simulink model "ASM1_Influentmodel"  (Simulink 7.6)
settings: Solver=ode45  StartTime=0.0  StopTime=728.0  RelTol=1e-6
undefined symbols (not defined in the file or in its folder): aHpercent, CODpart_gperPEperd, CODpart_HH_max, CODpart_HH_min, CODpart_HH_ns, CODpart_HH_nv, CODpart_HH_st, CODpart_Ind_kgperd, CODpart_Ind_max, CODpart_Ind_min, CODpart_Ind_ns, CODpart_Ind_nv, CODpart_Ind_st, CODsol_gperPEperd, CODsol_HH_max, CODsol_HH_min, CODsol_HH_ns, CODsol_HH_nv, CODsol_HH_st, CODsol_Ind_kgperd, CODsol_Ind_max, CODsol_Ind_min, CODsol_Ind_ns, CODsol_Ind_nv, CODsol_Ind_st, FFfraction, HHnoiseswitch, HHpolnoiseswitch, HHpopswitch, Indnoiseswitch, Indpolnoiseswitch, Indpopswitch, InfAmp, InfBias, Infcst, InfFreq, InfPhase, LLrain, PE, polnoiseswitch, Q_HH_ns, Q_HH_nv, Q_HH_st, Q_Ind_ns, Q_Ind_nv, Q_Ind_st, Q_SCI_ns, Q_SCI_nv, Q_SCI_st, QHHsatmax, QHHsatmin, QInd_weekday, QIndsatmax, QIndsatmin, Qpermm, QperPE, QSCIsatmax, QSCIsatmin, rain_nm, rain_ns ... (+85)
libraries: simulink x5
Description:
  | BSM2 influent model, version 15 March 2005
settings Model: Creator=Krist V. Gernaey  LastModifiedBy=xavier  ExtModeAutoUpdateStatusClock=off
settings DataIOCC: LimitDataPoints=off  SignalLoggingName=sigsOut  OutputOption=SpecifiedOutputTimes  OutputTimes=[119.0:1.0/96.0:728.0]
settings OptimizationCC: InitFltsAndDblsToZero=on
settings DebuggingCC: SaveWithParameterizedLinksMsg=none  SignalResolutionControl=TryResolveAllWithWarning  SolverPrmCheckMsg=none  MultiTaskDSMMsg=warning  MultiTaskCondExecSysMsg=none  StrictBusMsg=None
settings HardwareCC: TargetEndianess=LittleEndian  TargetHWDeviceType=MATLAB Host  ProdEqTarget=off
settings RTWCC: IncludeERTFirstTime=on

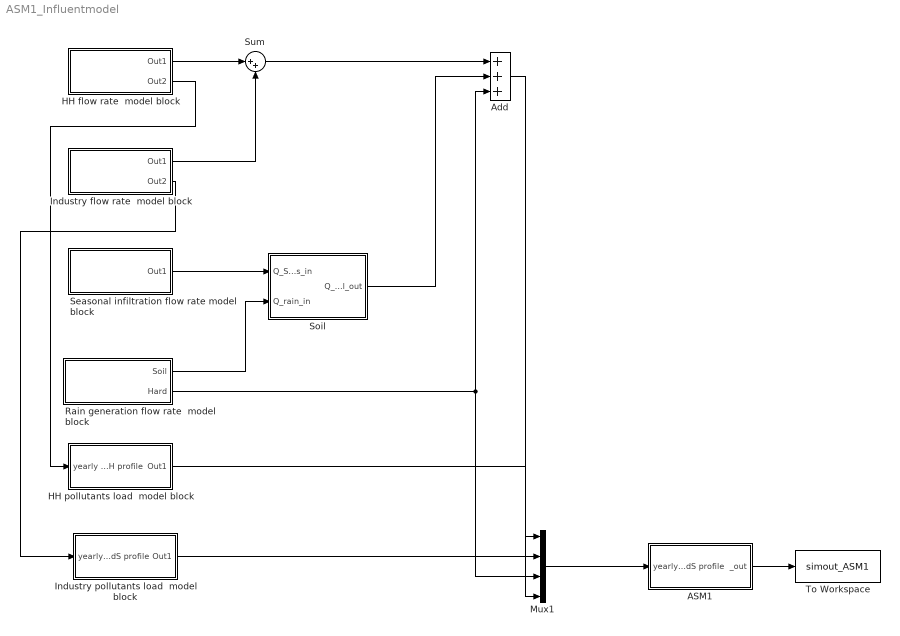
== system ASM1_Influentmodel ==
  ASM1 : Subsystem
  Add : Sum  Inputs=+++
  HH flow rate  model block : Subsystem
  "HH pollutants load  model block " : Subsystem
  Industry flow rate  model block : Subsystem
  "Industry pollutants load  model block " : Subsystem
  Mux1 : Mux
  Rain generation flow rate  model block : Subsystem
  Seasonal infiltration flow rate model block : Subsystem
  Soil : Subsystem
  Sum : Sum  Inputs=|++  SaturateOnIntegerOverflow=on
  To Workspace : ToWorkspace  VariableName=simout_ASM1  SampleTime=-1  SaveFormat=Array
  wires:
  Add/1 -> Mux1/4
  Rain generation flow rate  model block/2(Hard) -> Mux1/3, Add/3
  Soil/1(Q_Soil_out) -> Add/2
  Sum/1 -> Add/1
  HH flow rate  model block/1(Out1) -> Sum/1
  Rain generation flow rate  model block/1(Soil) -> Soil/2(Q_rain_in)
  Seasonal infiltration flow rate model block/1(Out1) -> Soil/1(Q_Seas_in)
  Industry flow rate  model block/1(Out1) -> Sum/2
  HH flow rate  model block/2(Out2) -> "HH pollutants load  model block "/1(yearly HH profile)
  Industry flow rate  model block/2(Out2) -> "Industry pollutants load  model block "/1(yearly_indS profile)
  "HH pollutants load  model block "/1(Out1) -> Mux1/1
  "Industry pollutants load  model block "/1(Out1) -> Mux1/2
  Mux1/1 -> ASM1/1(yearly_indS profile)
  ASM1/1(_out) -> To Workspace/1

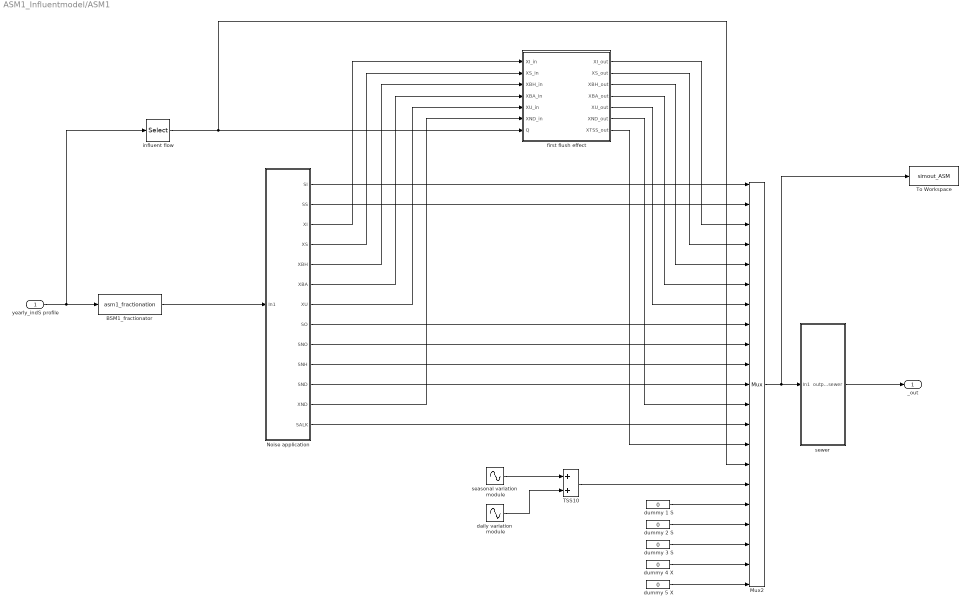
== system ASM1_Influentmodel/ASM1 ==
  yearly_indS profile : Inport
  BSM1_fractionator : S-Function  FunctionName=asm1_fractionation  Parameters=ASM1_PARS, ASM1_FRACTIONS  EnableBusSupport=off
  Mux2 : Mux  Inputs=21
  Noise application : Subsystem
  TSS10 : Sum
  To Workspace : ToWorkspace  VariableName=simout_ASM  SampleTime=-1  SaveFormat=Array
  daily variation  module : Sin  Amplitude=TdAmp  Bias=TdBias  Frequency=TdFreq  Phase=TdPhase  SampleTime=0
  dummy 1 S : Constant  Value=0
  dummy 2 S : Constant  Value=0
  dummy 3 S : Constant  Value=0
  dummy 4 X : Constant  Value=0
  dummy 5 X : Constant  Value=0
  first flush effect : Subsystem
  influent flow : Selector  InputPortWidth=12  IndexOptions=Index vector (dialog)  Indices=[12]  OutputSizes=1
  seasonal variation  module : Sin  Amplitude=TAmp  Bias=TBias  Frequency=TFreq  Phase=TPhase  SampleTime=0
  sewer : Subsystem
  _out : Outport
  wires:
  yearly_indS profile/1 -> influent flow/1, BSM1_fractionator/1
  BSM1_fractionator/1 -> Noise application/1(In1)
  Noise application/3(XI) -> first flush effect/1(XI_in)
  Noise application/4(XS) -> first flush effect/2(XS_in)
  Noise application/5(XBH) -> first flush effect/3(XBH_in)
  Noise application/6(XBA) -> first flush effect/4(XBA_in)
  Noise application/7(XU) -> first flush effect/5(XU_in)
  Noise application/12(XND) -> first flush effect/6(XND_in)
  influent flow/1 -> first flush effect/7(Q), Mux2/15
  Mux2/1 -> sewer/1(In1), To Workspace/1
  sewer/1(output sewer) -> _out/1
  dummy 5 X/1 -> Mux2/21
  dummy 4 X/1 -> Mux2/20
  dummy 3 S/1 -> Mux2/19
  dummy 2 S/1 -> Mux2/18
  dummy 1 S/1 -> Mux2/17
  Noise application/2(SS) -> Mux2/2
  Noise application/1(SI) -> Mux2/1
  first flush effect/1(XI_out) -> Mux2/3
  first flush effect/2(XS_out) -> Mux2/4
  first flush effect/3(XBH_out) -> Mux2/5
  first flush effect/4(XBA_out) -> Mux2/6
  first flush effect/5(XU_out) -> Mux2/7
  Noise application/8(SO) -> Mux2/8
  Noise application/9(SNO) -> Mux2/9
  Noise application/10(SNH) -> Mux2/10
  Noise application/11(SND) -> Mux2/11
  first flush effect/6(XND_out) -> Mux2/12
  Noise application/13(SALK) -> Mux2/13
  first flush effect/7(XTSS_out) -> Mux2/14
  seasonal variation  module/1 -> TSS10/1
  daily variation  module/1 -> TSS10/2
  TSS10/1 -> Mux2/16

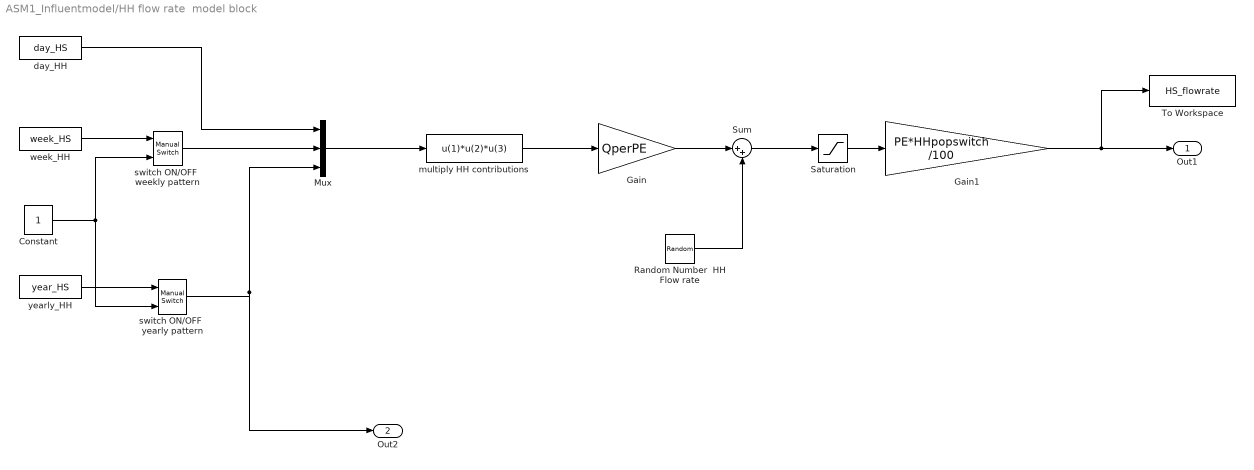
== system ASM1_Influentmodel/HH flow rate  model block ==
  Constant : Constant
  Gain : Gain  Gain=QperPE
  Gain1 : Gain  Gain=PE*HHpopswitch /100
  Mux : Mux  Inputs=3
  Random Number  HH Flow rate : RandomNumber  Variance=Q_HH_nv*HHnoiseswitch  Seed=Q_HH_ns  SampleTime=Q_HH_st
  Saturation : Saturate  UpperLimit=QHHsatmax  LowerLimit=QHHsatmin
  Sum : Sum  Inputs=|++
  To Workspace : ToWorkspace  VariableName=HS_flowrate  SampleTime=-1  SaveFormat=Array
  day_HH : FromWorkspace  VariableName=day_HS  SampleTime=1/24  Interpolate=off  OutputAfterFinalValue=Cyclic repetition
  multiply HH contributions : Fcn  Expr=u(1)*u(2)*u(3)
  switch ON/OFF  weekly pattern : simulink/Signal Routing/Manual Switch  SystemSampleTime=-1  sw=1  action=0  varsize=off
  switch ON/OFF  yearly pattern : simulink/Signal Routing/Manual Switch  SystemSampleTime=-1  sw=1  action=0  varsize=off
  week_HH : FromWorkspace  VariableName=week_HS  SampleTime=1  Interpolate=off  OutputAfterFinalValue=Cyclic repetition
  yearly_HH : FromWorkspace  VariableName=year_HS  SampleTime=1  Interpolate=off  OutputAfterFinalValue=Cyclic repetition
  Out1 : Outport
  Out2 : Outport  Port=2
  wires:
  multiply HH contributions/1 -> Gain/1
  Gain/1 -> Sum/1
  Saturation/1 -> Gain1/1
  Gain1/1 -> Out1/1, To Workspace/1
  Random Number  HH Flow rate/1 -> Sum/2
  week_HH/1 -> switch ON/OFF  weekly pattern/1
  yearly_HH/1 -> switch ON/OFF  yearly pattern/1
  day_HH/1 -> Mux/1
  switch ON/OFF  weekly pattern/1 -> Mux/2
  switch ON/OFF  yearly pattern/1 -> Mux/3, Out2/1
  Constant/1 -> switch ON/OFF  weekly pattern/2, switch ON/OFF  yearly pattern/2
  Mux/1 -> multiply HH contributions/1
  Sum/1 -> Saturation/1

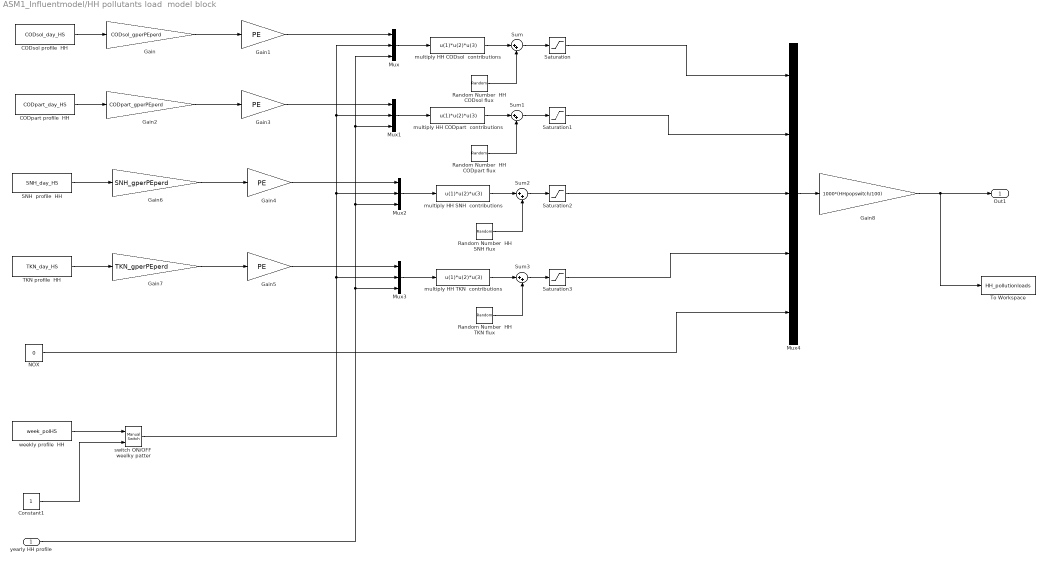
== system ASM1_Influentmodel/HH pollutants load  model block  ==
  yearly HH profile : Inport
  CODpart profile  HH : FromWorkspace  VariableName=CODpart_day_HS  SampleTime=1/24  Interpolate=off  OutputAfterFinalValue=Cyclic repetition
  CODsol profile  HH : FromWorkspace  VariableName=CODsol_day_HS  SampleTime=1/24  Interpolate=off  OutputAfterFinalValue=Cyclic repetition
  Constant1 : Constant
  Gain : Gain  Gain=CODsol_gperPEperd
  Gain{1,3..5} (4 alike) : Gain  Gain=PE
  Gain2 : Gain  Gain=CODpart_gperPEperd
  Gain6 : Gain  Gain=SNH_gperPEperd
  Gain7 : Gain  Gain=TKN_gperPEperd
  Gain8 : Gain  Gain=1000*(HHpopswitch/100)
  Mux{,1..3} (4 alike) : Mux  Inputs=3
  Mux4 : Mux  Inputs=5
  NOX : Constant  Value=0
  Random Number  HH CODpart flux : RandomNumber  Variance=CODpart_HH_nv*HHpolnoiseswitch  Seed=CODpart_HH_ns  SampleTime=CODpart_HH_st
  Random Number  HH CODsol flux : RandomNumber  Variance=CODsol_HH_nv*HHpolnoiseswitch  Seed=CODsol_HH_ns  SampleTime=CODsol_HH_st
  Random Number  HH SNH flux : RandomNumber  Variance=SNH_HH_nv*HHpolnoiseswitch  Seed=SNH_HH_ns  SampleTime=SNH_HH_st
  Random Number  HH TKN flux : RandomNumber  Variance=TKN_HH_nv*HHpolnoiseswitch  Seed=TKN_HH_ns  SampleTime=TKN_HH_st
  SNH  profile  HH : FromWorkspace  VariableName=SNH_day_HS  SampleTime=1/24  Interpolate=off  OutputAfterFinalValue=Cyclic repetition
  Saturation : Saturate  UpperLimit=CODsol_HH_max  LowerLimit=CODsol_HH_min
  Saturation1 : Saturate  UpperLimit=CODpart_HH_max  LowerLimit=CODpart_HH_min
  Saturation2 : Saturate  UpperLimit=SNH_HH_max  LowerLimit=SNH_HH_min
  Saturation3 : Saturate  UpperLimit=TKN_HH_max  LowerLimit=TKN_HH_min
  Sum{,1..3} (4 alike) : Sum  Inputs=|++
  TKN profile  HH : FromWorkspace  VariableName=TKN_day_HS  SampleTime=1/24  Interpolate=off  OutputAfterFinalValue=Cyclic repetition
  To Workspace : ToWorkspace  VariableName=HH_pollutionloads  SampleTime=-1  SaveFormat=Array
  multiply HH CODpart  contributions : Fcn  Expr=u(1)*u(2)*u(3)
  multiply HH CODsol  contributions : Fcn  Expr=u(1)*u(2)*u(3)
  multiply HH SNH  contributions : Fcn  Expr=u(1)*u(2)*u(3)
  multiply HH TKN  contributions : Fcn  Expr=u(1)*u(2)*u(3)
  switch ON/OFF  weelky patter : simulink/Signal Routing/Manual Switch  SystemSampleTime=-1  sw=1  action=0  varsize=off
  weekly profile  HH : FromWorkspace  VariableName=week_polHS  SampleTime=1  Interpolate=off  OutputAfterFinalValue=Cyclic repetition
  Out1 : Outport
  wires:
  Random Number  HH CODsol flux/1 -> Sum/2
  CODsol profile  HH/1 -> Gain/1
  Gain/1 -> Gain1/1
  Mux/1 -> multiply HH CODsol  contributions/1
  multiply HH CODsol  contributions/1 -> Sum/1
  Sum/1 -> Saturation/1
  Gain1/1 -> Mux/1
  Random Number  HH CODpart flux/1 -> Sum1/2
  CODpart profile  HH/1 -> Gain2/1
  Gain2/1 -> Gain3/1
  Mux1/1 -> multiply HH CODpart  contributions/1
  multiply HH CODpart  contributions/1 -> Sum1/1
  Sum1/1 -> Saturation1/1
  Gain3/1 -> Mux1/1
  Random Number  HH SNH flux/1 -> Sum2/2
  SNH  profile  HH/1 -> Gain6/1
  Gain6/1 -> Gain4/1
  Mux2/1 -> multiply HH SNH  contributions/1
  multiply HH SNH  contributions/1 -> Sum2/1
  Sum2/1 -> Saturation2/1
  Gain4/1 -> Mux2/1
  Random Number  HH TKN flux/1 -> Sum3/2
  TKN profile  HH/1 -> Gain7/1
  Gain7/1 -> Gain5/1
  Mux3/1 -> multiply HH TKN  contributions/1
  multiply HH TKN  contributions/1 -> Sum3/1
  Sum3/1 -> Saturation3/1
  Gain5/1 -> Mux3/1
  Mux4/1 -> Gain8/1
  Constant1/1 -> switch ON/OFF  weelky patter/2
  weekly profile  HH/1 -> switch ON/OFF  weelky patter/1
  Saturation/1 -> Mux4/1
  Saturation1/1 -> Mux4/2
  Saturation2/1 -> Mux4/3
  Saturation3/1 -> Mux4/4
  NOX/1 -> Mux4/5
  switch ON/OFF  weelky patter/1 -> Mux2/2, Mux/2, Mux1/2, Mux3/2
  yearly HH profile/1 -> Mux2/3, Mux/3, Mux1/3, Mux3/3
  Gain8/1 -> Out1/1, To Workspace/1

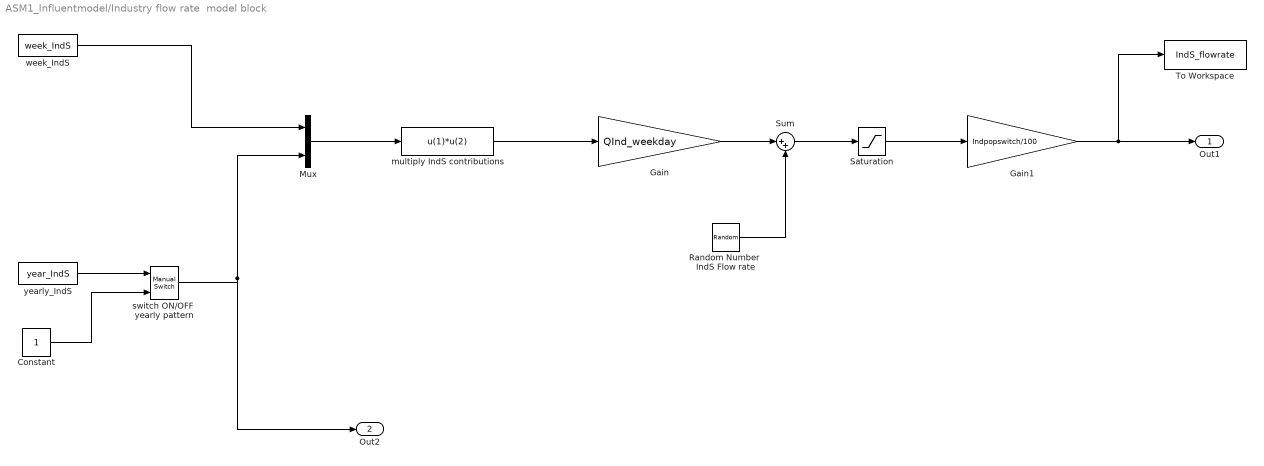
== system ASM1_Influentmodel/Industry flow rate  model block ==
  Constant : Constant
  Gain : Gain  Gain=QInd_weekday
  Gain1 : Gain  Gain=Indpopswitch/100
  Mux : Mux  Inputs=2
  Random Number  IndS Flow rate : RandomNumber  Variance=Q_Ind_nv*Indnoiseswitch  Seed=Q_Ind_ns  SampleTime=Q_Ind_st
  Saturation : Saturate  UpperLimit=QIndsatmax  LowerLimit=QIndsatmin
  Sum : Sum  Inputs=|++
  To Workspace : ToWorkspace  VariableName=IndS_flowrate  SampleTime=-1  SaveFormat=Array
  multiply IndS contributions : Fcn  Expr=u(1)*u(2)
  switch ON/OFF  yearly pattern : simulink/Signal Routing/Manual Switch  SystemSampleTime=-1  sw=1  action=0  varsize=off
  week_IndS : FromWorkspace  VariableName=week_IndS  SampleTime=1/6  Interpolate=off  OutputAfterFinalValue=Cyclic repetition
  yearly_IndS : FromWorkspace  VariableName=year_IndS  SampleTime=1  Interpolate=off  OutputAfterFinalValue=Cyclic repetition
  Out1 : Outport
  Out2 : Outport  Port=2
  wires:
  multiply IndS contributions/1 -> Gain/1
  Gain/1 -> Sum/1
  Sum/1 -> Saturation/1
  Saturation/1 -> Gain1/1
  Gain1/1 -> Out1/1, To Workspace/1
  Random Number  IndS Flow rate/1 -> Sum/2
  yearly_IndS/1 -> switch ON/OFF  yearly pattern/1
  week_IndS/1 -> Mux/1
  switch ON/OFF  yearly pattern/1 -> Mux/2, Out2/1
  Constant/1 -> switch ON/OFF  yearly pattern/2
  Mux/1 -> multiply IndS contributions/1

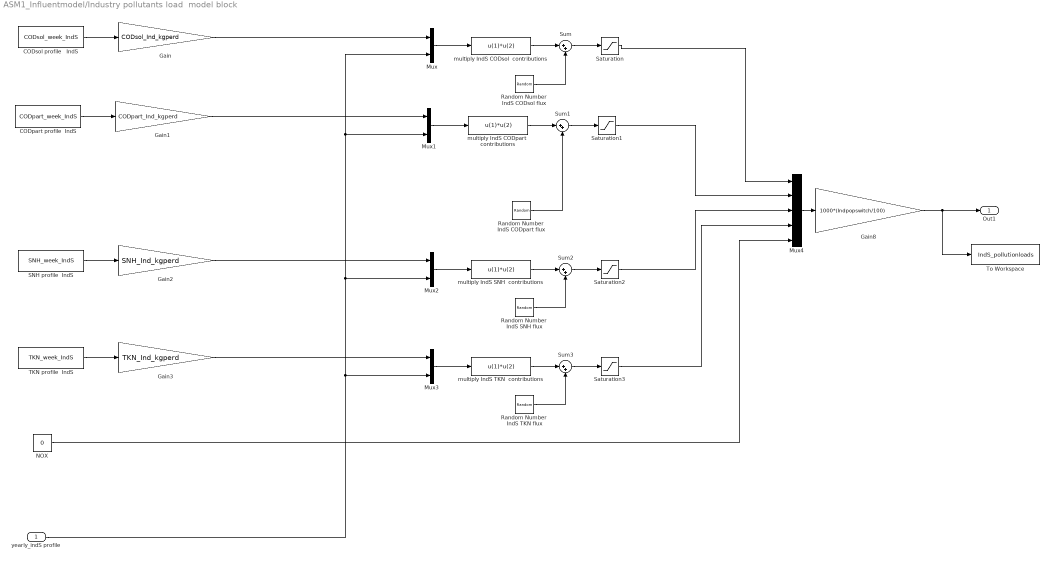
== system ASM1_Influentmodel/Industry pollutants load  model block  ==
  yearly_indS profile : Inport
  CODpart profile  IndS : FromWorkspace  VariableName=CODpart_week_IndS  SampleTime=1/6  Interpolate=off  OutputAfterFinalValue=Cyclic repetition
  CODsol profile   IndS : FromWorkspace  VariableName=CODsol_week_IndS  SampleTime=1/6  Interpolate=off  OutputAfterFinalValue=Cyclic repetition
  Gain : Gain  Gain=CODsol_Ind_kgperd
  Gain1 : Gain  Gain=CODpart_Ind_kgperd
  Gain2 : Gain  Gain=SNH_Ind_kgperd
  Gain3 : Gain  Gain=TKN_Ind_kgperd
  Gain8 : Gain  Gain=1000*(Indpopswitch/100)
  Mux{,1..3} (4 alike) : Mux  Inputs=2
  Mux4 : Mux  Inputs=5
  NOX : Constant  Value=0
  Random Number  IndS CODpart flux : RandomNumber  Variance=CODpart_Ind_nv*Indpolnoiseswitch  Seed=CODpart_Ind_ns  SampleTime=CODpart_Ind_st
  Random Number  IndS CODsol flux : RandomNumber  Variance=CODsol_Ind_nv*Indpolnoiseswitch  Seed=CODsol_Ind_ns  SampleTime=CODsol_Ind_st
  Random Number  IndS SNH flux : RandomNumber  Variance=SNH_Ind_nv*Indpolnoiseswitch  Seed=SNH_Ind_ns  SampleTime=SNH_Ind_st
  Random Number  IndS TKN flux : RandomNumber  Variance=TKN_Ind_nv*Indpolnoiseswitch  Seed=TKN_Ind_ns  SampleTime=TKN_Ind_st
  SNH profile  IndS : FromWorkspace  VariableName=SNH_week_IndS  SampleTime=1/6  Interpolate=off  OutputAfterFinalValue=Cyclic repetition
  Saturation : Saturate  UpperLimit=CODsol_Ind_max  LowerLimit=CODsol_Ind_min
  Saturation1 : Saturate  UpperLimit=CODpart_Ind_max  LowerLimit=CODpart_Ind_min
  Saturation2 : Saturate  UpperLimit=SNH_Ind_max  LowerLimit=SNH_Ind_min
  Saturation3 : Saturate  UpperLimit=TKN_Ind_max  LowerLimit=TKN_Ind_min
  Sum{,1..3} (4 alike) : Sum  Inputs=|++
  TKN profile  IndS : FromWorkspace  VariableName=TKN_week_IndS  SampleTime=1/6  Interpolate=off  OutputAfterFinalValue=Cyclic repetition
  To Workspace : ToWorkspace  VariableName=IndS_pollutionloads  SampleTime=-1  SaveFormat=Array
  multiply IndS CODpart  contributions : Fcn  Expr=u(1)*u(2)
  multiply IndS CODsol  contributions : Fcn  Expr=u(1)*u(2)
  multiply IndS SNH  contributions : Fcn  Expr=u(1)*u(2)
  multiply IndS TKN  contributions : Fcn  Expr=u(1)*u(2)
  Out1 : Outport
  wires:
  Random Number  IndS CODsol flux/1 -> Sum/2
  CODsol profile   IndS/1 -> Gain/1
  Mux/1 -> multiply IndS CODsol  contributions/1
  multiply IndS CODsol  contributions/1 -> Sum/1
  Sum/1 -> Saturation/1
  Mux4/1 -> Gain8/1
  Gain/1 -> Mux/1
  Random Number  IndS CODpart flux/1 -> Sum1/2
  CODpart profile  IndS/1 -> Gain1/1
  Mux1/1 -> multiply IndS CODpart  contributions/1
  multiply IndS CODpart  contributions/1 -> Sum1/1
  Sum1/1 -> Saturation1/1
  Gain1/1 -> Mux1/1
  Random Number  IndS SNH flux/1 -> Sum2/2
  SNH profile  IndS/1 -> Gain2/1
  Mux2/1 -> multiply IndS SNH  contributions/1
  multiply IndS SNH  contributions/1 -> Sum2/1
  Sum2/1 -> Saturation2/1
  Gain2/1 -> Mux2/1
  Random Number  IndS TKN flux/1 -> Sum3/2
  TKN profile  IndS/1 -> Gain3/1
  Mux3/1 -> multiply IndS TKN  contributions/1
  multiply IndS TKN  contributions/1 -> Sum3/1
  Sum3/1 -> Saturation3/1
  Gain3/1 -> Mux3/1
  yearly_indS profile/1 -> Mux3/2, Mux2/2, Mux/2, Mux1/2
  Saturation/1 -> Mux4/1
  Saturation1/1 -> Mux4/2
  Saturation2/1 -> Mux4/3
  Saturation3/1 -> Mux4/4
  NOX/1 -> Mux4/5
  Gain8/1 -> Out1/1, To Workspace/1

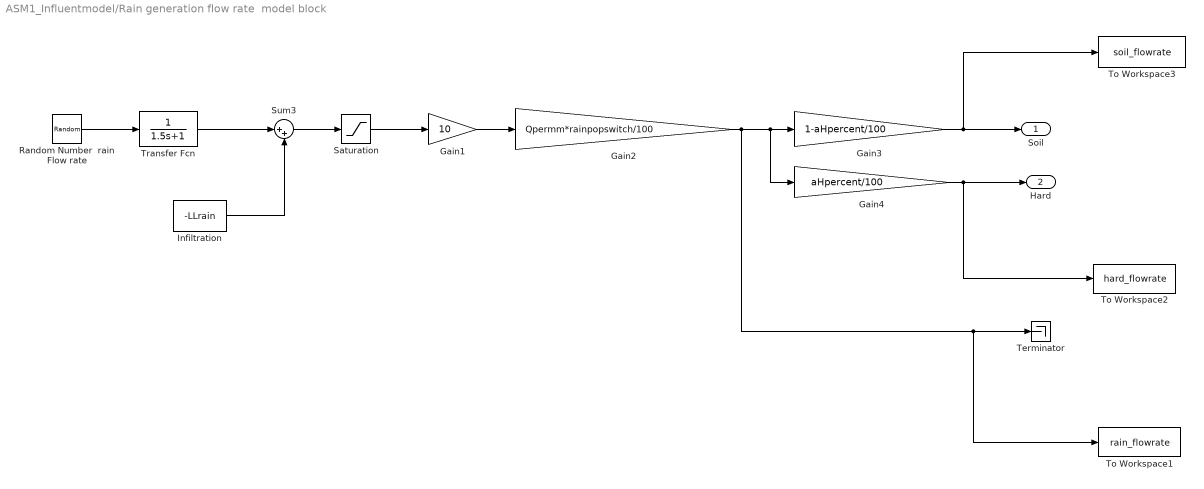
== system ASM1_Influentmodel/Rain generation flow rate  model block ==
  Gain1 : Gain  Gain=10  SaturateOnIntegerOverflow=on  OutDataTypeStr=Inherit: Same as input  ParamDataTypeStr=Inherit: Same as input
  Gain2 : Gain  Gain=Qpermm*rainpopswitch/100  SaturateOnIntegerOverflow=on  OutDataTypeStr=Inherit: Same as input  ParamDataTypeStr=Inherit: Same as input
  Gain3 : Gain  Gain=1-aHpercent/100  SaturateOnIntegerOverflow=on  OutDataTypeStr=Inherit: Same as input  ParamDataTypeStr=Inherit: Same as input
  Gain4 : Gain  Gain=aHpercent/100  SaturateOnIntegerOverflow=on  OutDataTypeStr=Inherit: Same as input  ParamDataTypeStr=Inherit: Same as input
  Infiltration : Constant  Value=-LLrain
  Random Number  rain Flow rate : RandomNumber  Mean=rain_nm  Variance=rain_nv  Seed=rain_ns  SampleTime=rain_st
  Saturation : Saturate  UpperLimit=rainmax  LowerLimit=rainmin
  Sum3 : Sum  Inputs=|++  SaturateOnIntegerOverflow=on
  Terminator : Terminator
  To Workspace1 : ToWorkspace  VariableName=rain_flowrate  SampleTime=-1  SaveFormat=Array
  To Workspace2 : ToWorkspace  VariableName=hard_flowrate  SampleTime=-1  SaveFormat=Array
  To Workspace3 : ToWorkspace  VariableName=soil_flowrate  SampleTime=-1  SaveFormat=Array
  Transfer Fcn : TransferFcn  Denominator=[1.5 1]
  Soil : Outport
  Hard : Outport  Port=2
  wires:
  Random Number  rain Flow rate/1 -> Transfer Fcn/1
  Gain3/1 -> Soil/1, To Workspace3/1
  Gain4/1 -> Hard/1, To Workspace2/1
  Gain2/1 -> Gain4/1, Gain3/1, To Workspace1/1, Terminator/1
  Gain1/1 -> Gain2/1
  Saturation/1 -> Gain1/1
  Infiltration/1 -> Sum3/2
  Transfer Fcn/1 -> Sum3/1
  Sum3/1 -> Saturation/1

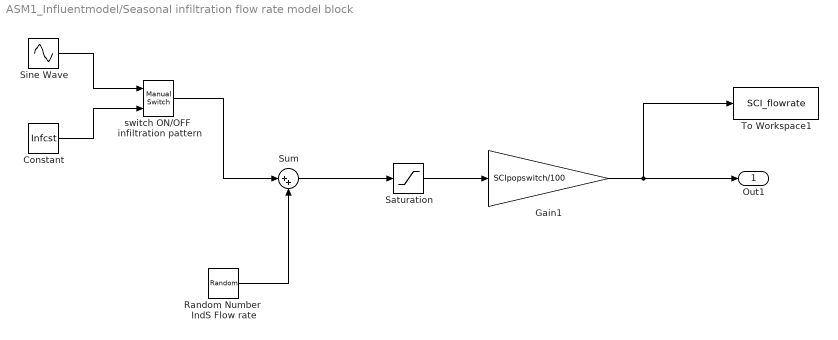
== system ASM1_Influentmodel/Seasonal infiltration flow rate model block ==
  Constant : Constant  Value=Infcst
  Gain1 : Gain  Gain=SCIpopswitch/100
  Random Number  IndS Flow rate : RandomNumber  Variance=Q_SCI_nv*SCInoiseswitch  Seed=Q_SCI_ns  SampleTime=Q_SCI_st
  Saturation : Saturate  UpperLimit=QSCIsatmax  LowerLimit=QSCIsatmin
  Sine Wave : Sin  Amplitude=InfAmp  Bias=InfBias  Frequency=InfFreq  Phase=InfPhase  SampleTime=0
  Sum : Sum  Inputs=|++
  To Workspace1 : ToWorkspace  VariableName=SCI_flowrate  SampleTime=-1  SaveFormat=Array
  switch ON/OFF  infiltration pattern : simulink/Signal Routing/Manual Switch  SystemSampleTime=-1  sw=1  action=0  varsize=off
  Out1 : Outport
  wires:
  switch ON/OFF  infiltration pattern/1 -> Sum/1
  Sum/1 -> Saturation/1
  Saturation/1 -> Gain1/1
  Gain1/1 -> Out1/1, To Workspace1/1
  Random Number  IndS Flow rate/1 -> Sum/2
  Sine Wave/1 -> switch ON/OFF  infiltration pattern/1
  Constant/1 -> switch ON/OFF  infiltration pattern/2

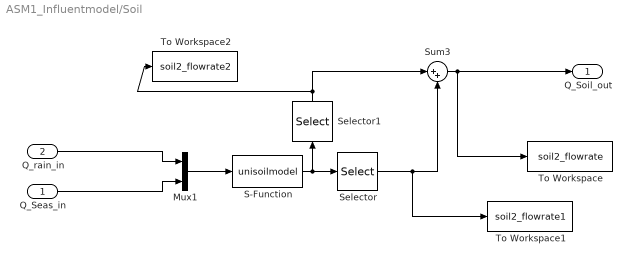
== system ASM1_Influentmodel/Soil ==
  Q_Seas_in : Inport
  Q_rain_in : Inport  Port=2
  Mux1 : Mux  Inputs=2
  S-Function : S-Function  FunctionName=unisoilmodel  Parameters=XINITSOIL, PARS_SOIL  EnableBusSupport=off
  Selector : Selector  InputPortWidth=4  IndexOptions=Index vector (dialog)  Indices=[1]  OutputSizes=1
  Selector1 : Selector  InputPortWidth=4  IndexOptions=Index vector (dialog)  Indices=[2]  OutputSizes=1
  Sum3 : Sum  Inputs=|++  SaturateOnIntegerOverflow=on
  To Workspace : ToWorkspace  VariableName=soil2_flowrate  SampleTime=-1  SaveFormat=Array
  To Workspace1 : ToWorkspace  VariableName=soil2_flowrate1  SampleTime=-1  SaveFormat=Array
  To Workspace2 : ToWorkspace  VariableName=soil2_flowrate2  SampleTime=-1  SaveFormat=Array
  Q_Soil_out : Outport
  wires:
  S-Function/1 -> Selector/1, Selector1/1
  Selector1/1 -> Sum3/1, To Workspace2/1
  Selector/1 -> Sum3/2, To Workspace1/1
  Sum3/1 -> Q_Soil_out/1, To Workspace/1
  Mux1/1 -> S-Function/1
  Q_rain_in/1 -> Mux1/1
  Q_Seas_in/1 -> Mux1/2

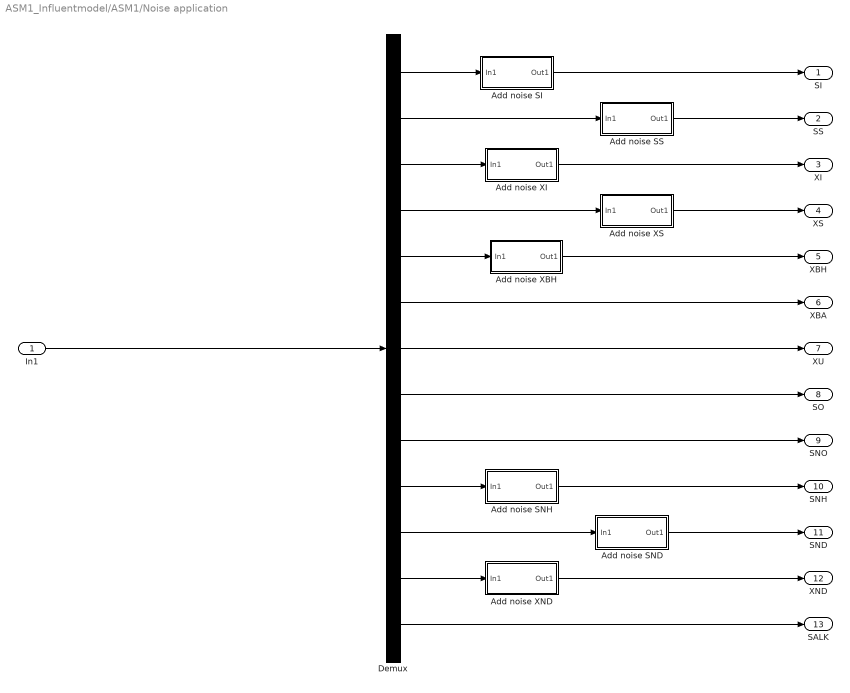
== system ASM1_Influentmodel/ASM1/Noise application ==
  In1 : Inport
  Add noise SI : Subsystem
  Add noise SND : Subsystem
  Add noise SNH : Subsystem
  Add noise SS : Subsystem
  Add noise XBH : Subsystem
  Add noise XI : Subsystem
  Add noise XND : Subsystem
  Add noise XS : Subsystem
  Demux : Demux  Outputs=[1 1 1 1 1 1 1 1 1 1 1 1 1]
  SI : Outport
  SS : Outport  Port=2
  XI : Outport  Port=3
  XS : Outport  Port=4
  XBH : Outport  Port=5
  XBA : Outport  Port=6
  XU : Outport  Port=7
  SO : Outport  Port=8
  SNO : Outport  Port=9
  SNH : Outport  Port=10
  SND : Outport  Port=11
  XND : Outport  Port=12
  SALK : Outport  Port=13
  wires:
  In1/1 -> Demux/1
  Demux/1 -> Add noise SI/1(In1)
  Demux/2 -> Add noise SS/1(In1)
  Demux/3 -> Add noise XI/1(In1)
  Demux/4 -> Add noise XS/1(In1)
  Demux/5 -> Add noise XBH/1(In1)
  Demux/6 -> XBA/1
  Demux/7 -> XU/1
  Demux/8 -> SO/1
  Demux/9 -> SNO/1
  Demux/10 -> Add noise SNH/1(In1)
  Demux/11 -> Add noise SND/1(In1)
  Demux/12 -> Add noise XND/1(In1)
  Demux/13 -> SALK/1
  Add noise SI/1(Out1) -> SI/1
  Add noise SS/1(Out1) -> SS/1
  Add noise XI/1(Out1) -> XI/1
  Add noise XS/1(Out1) -> XS/1
  Add noise XBH/1(Out1) -> XBH/1
  Add noise SNH/1(Out1) -> SNH/1
  Add noise SND/1(Out1) -> SND/1
  Add noise XND/1(Out1) -> XND/1

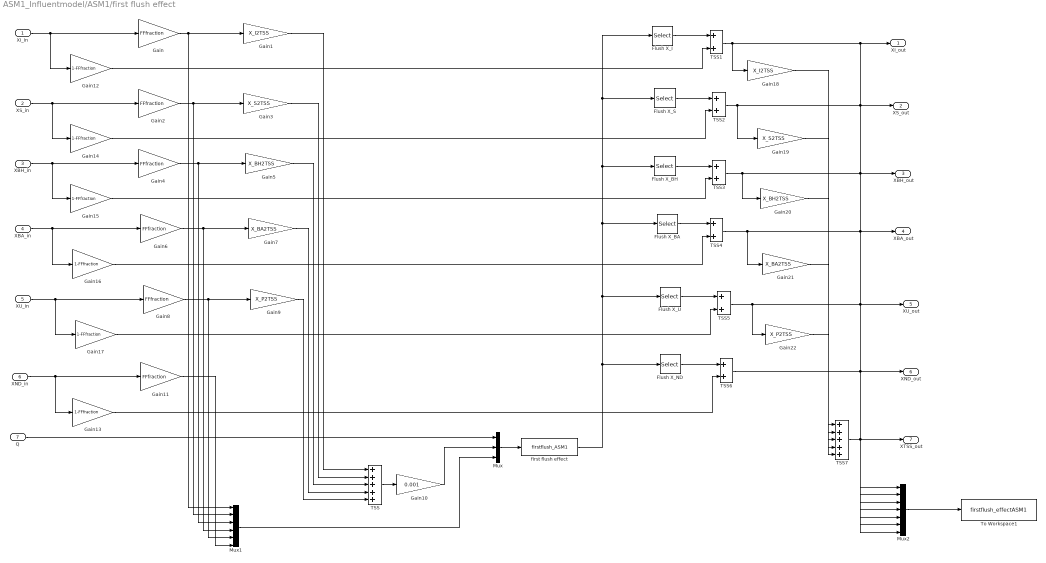
== system ASM1_Influentmodel/ASM1/first flush effect ==
  XI_in : Inport
  XS_in : Inport  Port=2
  XBH_in : Inport  Port=3
  XBA_in : Inport  Port=4
  XU_in : Inport  Port=5
  XND_in : Inport  Port=6
  Q : Inport  Port=7
  Flush X_BA : Selector  InputPortWidth=15  IndexOptions=Index vector (dialog)  Indices=[6]  OutputSizes=1
  Flush X_BH : Selector  InputPortWidth=15  IndexOptions=Index vector (dialog)  Indices=[5]  OutputSizes=1
  Flush X_I : Selector  InputPortWidth=15  IndexOptions=Index vector (dialog)  Indices=[3]  OutputSizes=1
  Flush X_ND : Selector  InputPortWidth=15  IndexOptions=Index vector (dialog)  Indices=[8]  OutputSizes=1
  Flush X_S : Selector  InputPortWidth=15  IndexOptions=Index vector (dialog)  Indices=[4]  OutputSizes=1
  Flush X_U : Selector  InputPortWidth=15  IndexOptions=Index vector (dialog)  Indices=[7]  OutputSizes=1
  Gain{,2,4,6,8,11} (6 alike) : Gain  Gain=FFfraction
  Gain1 : Gain  Gain=X_I2TSS
  Gain10 : Gain  Gain=0.001
  Gain{12..17} (6 alike) : Gain  Gain=1-FFfraction
  Gain18 : Gain  Gain=X_I2TSS
  Gain19 : Gain  Gain=X_S2TSS
  Gain20 : Gain  Gain=X_BH2TSS
  Gain21 : Gain  Gain=X_BA2TSS
  Gain22 : Gain  Gain=X_P2TSS
  Gain3 : Gain  Gain=X_S2TSS
  Gain5 : Gain  Gain=X_BH2TSS
  Gain7 : Gain  Gain=X_BA2TSS
  Gain9 : Gain  Gain=X_P2TSS
  Mux : Mux  Inputs=3
  Mux1 : Mux  Inputs=6
  Mux2 : Mux  Inputs=7
  TSS : Sum  Inputs=+++++
  TSS{1..6} (6 alike) : Sum
  TSS7 : Sum  Inputs=+++++
  To Workspace1 : ToWorkspace  VariableName=firstflush_effectASM1  SampleTime=-1  SaveFormat=Array
  first flush effect : S-Function  FunctionName=firstflush_ASM1  Parameters=ASM1_XINIT, SSPARS  EnableBusSupport=off
  XI_out : Outport
  XS_out : Outport  Port=2
  XBH_out : Outport  Port=3
  XBA_out : Outport  Port=4
  XU_out : Outport  Port=5
  XND_out : Outport  Port=6
  XTSS_out : Outport  Port=7
  wires:
  XI_in/1 -> Gain/1, Gain12/1
  Gain/1 -> Gain1/1, Mux1/1
  XS_in/1 -> Gain2/1, Gain14/1
  Gain2/1 -> Gain3/1, Mux1/2
  XBH_in/1 -> Gain4/1, Gain15/1
  Gain4/1 -> Gain5/1, Mux1/3
  XBA_in/1 -> Gain6/1, Gain16/1
  Gain6/1 -> Gain7/1, Mux1/4
  XU_in/1 -> Gain8/1, Gain17/1
  Gain8/1 -> Gain9/1, Mux1/5
  Gain1/1 -> TSS/1
  Gain3/1 -> TSS/2
  Gain5/1 -> TSS/3
  Gain7/1 -> TSS/4
  Gain9/1 -> TSS/5
  Mux1/1 -> Mux/3
  Gain11/1 -> Mux1/6
  XND_in/1 -> Gain11/1, Gain13/1
  Q/1 -> Mux/1
  Mux/1 -> first flush effect/1
  TSS/1 -> Gain10/1
  Gain10/1 -> Mux/2
  Gain12/1 -> TSS1/2
  first flush effect/1 -> Flush X_I/1, Flush X_S/1, Flush X_BH/1, Flush X_BA/1, Flush X_U/1, Flush X_ND/1
  Flush X_I/1 -> TSS1/1
  Flush X_S/1 -> TSS2/1
  Gain14/1 -> TSS2/2
  Flush X_BH/1 -> TSS3/1
  Gain15/1 -> TSS3/2
  Gain16/1 -> TSS4/2
  Flush X_BA/1 -> TSS4/1
  Gain17/1 -> TSS5/2
  Flush X_U/1 -> TSS5/1
  Gain13/1 -> TSS6/2
  Flush X_ND/1 -> TSS6/1
  TSS1/1 -> Gain18/1, XI_out/1, Mux2/1
  TSS2/1 -> Gain19/1, XS_out/1, Mux2/2
  TSS3/1 -> Gain20/1, XBH_out/1, Mux2/3
  TSS4/1 -> Gain21/1, XBA_out/1, Mux2/4
  TSS5/1 -> Gain22/1, XU_out/1, Mux2/5
  TSS6/1 -> XND_out/1, Mux2/6
  Gain18/1 -> TSS7/1
  Gain19/1 -> TSS7/2
  Gain20/1 -> TSS7/3
  Gain21/1 -> TSS7/4
  Gain22/1 -> TSS7/5
  TSS7/1 -> XTSS_out/1, Mux2/7
  Mux2/1 -> To Workspace1/1

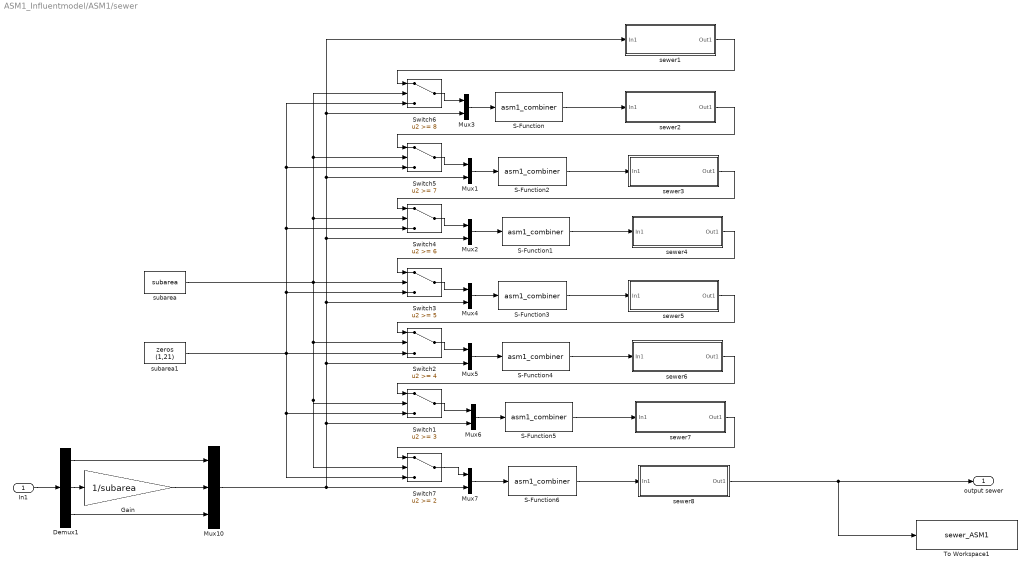
== system ASM1_Influentmodel/ASM1/sewer ==
  In1 : Inport
  Demux1 : Demux  Outputs=[14 1 6]
  Gain : Gain  Gain=1/subarea
  Mux{1..7} (7 alike) : Mux  Inputs=2
  Mux10 : Mux  Inputs=3
  S-Function{,1..6} (7 alike) : S-Function  FunctionName=asm1_combiner  EnableBusSupport=off
  Switch1 : Switch  Threshold=3  SaturateOnIntegerOverflow=on
  Switch2 : Switch  Threshold=4  SaturateOnIntegerOverflow=on
  Switch3 : Switch  Threshold=5  SaturateOnIntegerOverflow=on
  Switch4 : Switch  Threshold=6  SaturateOnIntegerOverflow=on
  Switch5 : Switch  Threshold=7  SaturateOnIntegerOverflow=on
  Switch6 : Switch  Threshold=8  SaturateOnIntegerOverflow=on
  Switch7 : Switch  Threshold=2  SaturateOnIntegerOverflow=on
  To Workspace1 : ToWorkspace  VariableName=sewer_ASM1  SampleTime=-1  SaveFormat=Array
  sewer1 : Subsystem
  sewer2 : Subsystem
  sewer3 : Subsystem
  sewer4 : Subsystem
  sewer5 : Subsystem
  sewer6 : Subsystem
  sewer7 : Subsystem
  sewer8 : Subsystem
  subarea : Constant  Value=subarea
  subarea1 : Constant  Value=zeros (1,21)
  output sewer : Outport
  wires:
  In1/1 -> Demux1/1
  Demux1/2 -> Gain/1
  Demux1/1 -> Mux10/1
  Demux1/3 -> Mux10/3
  Gain/1 -> Mux10/2
  S-Function/1 -> sewer2/1(In1)
  sewer2/1(Out1) -> Switch5/1
  S-Function2/1 -> sewer3/1(In1)
  sewer3/1(Out1) -> Switch4/1
  S-Function1/1 -> sewer4/1(In1)
  sewer4/1(Out1) -> Switch3/1
  S-Function3/1 -> sewer5/1(In1)
  sewer5/1(Out1) -> Switch2/1
  sewer1/1(Out1) -> Switch6/1
  S-Function4/1 -> sewer6/1(In1)
  sewer6/1(Out1) -> Switch1/1
  S-Function5/1 -> sewer7/1(In1)
  sewer7/1(Out1) -> Switch7/1
  S-Function6/1 -> sewer8/1(In1)
  Mux10/1 -> Mux1/2, Mux3/2, sewer1/1(In1), Mux2/2, Mux4/2, Mux5/2, Mux6/2, Mux7/2
  Switch6/1 -> Mux3/1
  Mux3/1 -> S-Function/1
  Switch5/1 -> Mux1/1
  Switch4/1 -> Mux2/1
  Switch3/1 -> Mux4/1
  Switch1/1 -> Mux6/1
  Switch2/1 -> Mux5/1
  Switch7/1 -> Mux7/1
  Mux1/1 -> S-Function2/1
  Mux2/1 -> S-Function1/1
  Mux4/1 -> S-Function3/1
  Mux5/1 -> S-Function4/1
  Mux6/1 -> S-Function5/1
  Mux7/1 -> S-Function6/1
  sewer8/1(Out1) -> output sewer/1, To Workspace1/1
  subarea/1 -> Switch3/2, Switch6/2, Switch5/2, Switch4/2, Switch2/2, Switch7/2, Switch1/2
  subarea1/1 -> Switch2/3, Switch6/3, Switch5/3, Switch4/3, Switch3/3, Switch1/3, Switch7/3

== system ASM1_Influentmodel/ASM1/Noise application/Add noise SI ==
  In1 : Inport
  Random Number : RandomNumber  Variance=SI_nv*polnoiseswitch  Seed=SI_ns  SampleTime=SI_st
  Saturation : Saturate  UpperLimit=SI_max  LowerLimit=SI_min
  Sum : Sum  Inputs=|++  SaturateOnIntegerOverflow=on
  Out1 : Outport
  wires:
  Sum/1 -> Saturation/1
  Random Number/1 -> Sum/2
  Saturation/1 -> Out1/1
  In1/1 -> Sum/1

== system ASM1_Influentmodel/ASM1/Noise application/Add noise SND ==
  In1 : Inport
  Random Number : RandomNumber  Variance=SND_nv*polnoiseswitch  Seed=SND_ns  SampleTime=SND_st
  Saturation : Saturate  UpperLimit=SND_max  LowerLimit=SND_min
  Sum : Sum  Inputs=|++  SaturateOnIntegerOverflow=on
  Out1 : Outport
  wires:
  Sum/1 -> Saturation/1
  Random Number/1 -> Sum/2
  Saturation/1 -> Out1/1
  In1/1 -> Sum/1

== system ASM1_Influentmodel/ASM1/Noise application/Add noise SNH ==
  In1 : Inport
  Random Number : RandomNumber  Variance=SNH_nv*polnoiseswitch  Seed=SNH_ns  SampleTime=SNH_st
  Saturation : Saturate  UpperLimit=SNH_max  LowerLimit=SNH_min
  Sum : Sum  Inputs=|++  SaturateOnIntegerOverflow=on
  Out1 : Outport
  wires:
  Sum/1 -> Saturation/1
  Random Number/1 -> Sum/2
  Saturation/1 -> Out1/1
  In1/1 -> Sum/1

== system ASM1_Influentmodel/ASM1/Noise application/Add noise SS ==
  In1 : Inport
  Random Number : RandomNumber  Variance=SS_nv*polnoiseswitch  Seed=SS_ns  SampleTime=SS_st
  Saturation : Saturate  UpperLimit=SS_max  LowerLimit=SS_min
  Sum : Sum  Inputs=|++  SaturateOnIntegerOverflow=on
  Out1 : Outport
  wires:
  Sum/1 -> Saturation/1
  Random Number/1 -> Sum/2
  Saturation/1 -> Out1/1
  In1/1 -> Sum/1

== system ASM1_Influentmodel/ASM1/Noise application/Add noise XBH ==
  In1 : Inport
  Random Number : RandomNumber  Variance=XBH_nv*polnoiseswitch  Seed=XBH_ns  SampleTime=XBH_st
  Saturation : Saturate  UpperLimit=XBH_max  LowerLimit=XBH_min
  Sum : Sum  Inputs=|++  SaturateOnIntegerOverflow=on
  Out1 : Outport
  wires:
  Sum/1 -> Saturation/1
  Random Number/1 -> Sum/2
  Saturation/1 -> Out1/1
  In1/1 -> Sum/1

== system ASM1_Influentmodel/ASM1/Noise application/Add noise XI ==
  In1 : Inport
  Random Number : RandomNumber  Variance=XI_nv*polnoiseswitch  Seed=XI_ns  SampleTime=XI_st
  Saturation : Saturate  UpperLimit=XI_max  LowerLimit=XI_min
  Sum : Sum  Inputs=|++  SaturateOnIntegerOverflow=on
  Out1 : Outport
  wires:
  Sum/1 -> Saturation/1
  Random Number/1 -> Sum/2
  Saturation/1 -> Out1/1
  In1/1 -> Sum/1

== system ASM1_Influentmodel/ASM1/Noise application/Add noise XND ==
  In1 : Inport
  Random Number : RandomNumber  Variance=XND_nv*polnoiseswitch  Seed=XND_ns  SampleTime=XND_st
  Saturation : Saturate  UpperLimit=XND_max  LowerLimit=XND_min
  Sum : Sum  Inputs=|++  SaturateOnIntegerOverflow=on
  Out1 : Outport
  wires:
  Sum/1 -> Saturation/1
  Random Number/1 -> Sum/2
  Saturation/1 -> Out1/1
  In1/1 -> Sum/1

== system ASM1_Influentmodel/ASM1/Noise application/Add noise XS ==
  In1 : Inport
  Random Number : RandomNumber  Variance=XS_nv*polnoiseswitch  Seed=XS_ns  SampleTime=XS_st
  Saturation : Saturate  UpperLimit=XS_max  LowerLimit=XS_min
  Sum : Sum  Inputs=|++  SaturateOnIntegerOverflow=on
  Out1 : Outport
  wires:
  Sum/1 -> Saturation/1
  Random Number/1 -> Sum/2
  Saturation/1 -> Out1/1
  In1/1 -> Sum/1

== system ASM1_Influentmodel/ASM1/sewer/sewer1 ==
  In1 : Inport
  Constant : Constant
  Mux1 : Mux  Inputs=2
  S-Function : S-Function  FunctionName=sewer_asm1  Parameters=ASM1_SEWERINIT, ASM1_PARS, SPAR  EnableBusSupport=off
  S-Function1 : S-Function  FunctionName=sewer_asm1  Parameters=ASM1_SEWERINIT, ASM1_PARS, SPAR  EnableBusSupport=off
  S-Function2 : S-Function  FunctionName=sewer_asm1  Parameters=ASM1_SEWERINIT, ASM1_PARS, SPAR  EnableBusSupport=off
  Selector9 : Selector  InputPortWidth=22  IndexOptions=Index vector (dialog)  Indices=[1 2 3 4 5 6 7 8 9 10 11 12 13 14 15 16 17 18 19 20 21]  OutputSizes=1
  Out1 : Outport
  wires:
  S-Function/1 -> S-Function1/1
  S-Function1/1 -> S-Function2/1
  S-Function2/1 -> Selector9/1
  Mux1/1 -> S-Function/1
  Constant/1 -> Mux1/2
  In1/1 -> Mux1/1
  Selector9/1 -> Out1/1

== system ASM1_Influentmodel/ASM1/sewer/sewer2 ==
  In1 : Inport
  Constant : Constant
  Mux1 : Mux  Inputs=2
  S-Function : S-Function  FunctionName=sewer_asm1  Parameters=ASM1_SEWERINIT, ASM1_PARS, SPAR  EnableBusSupport=off
  S-Function1 : S-Function  FunctionName=sewer_asm1  Parameters=ASM1_SEWERINIT, ASM1_PARS, SPAR  EnableBusSupport=off
  S-Function2 : S-Function  FunctionName=sewer_asm1  Parameters=ASM1_SEWERINIT, ASM1_PARS, SPAR  EnableBusSupport=off
  Selector9 : Selector  InputPortWidth=22  IndexOptions=Index vector (dialog)  Indices=[1 2 3 4 5 6 7 8 9 10 11 12 13 14 15 16 17 18 19 20 21]  OutputSizes=1
  Out1 : Outport
  wires:
  S-Function/1 -> S-Function1/1
  S-Function1/1 -> S-Function2/1
  S-Function2/1 -> Selector9/1
  Mux1/1 -> S-Function/1
  Constant/1 -> Mux1/2
  Selector9/1 -> Out1/1
  In1/1 -> Mux1/1

== system ASM1_Influentmodel/ASM1/sewer/sewer3 ==
  In1 : Inport
  Constant : Constant
  Mux1 : Mux  Inputs=2
  S-Function : S-Function  FunctionName=sewer_asm1  Parameters=ASM1_SEWERINIT, ASM1_PARS, SPAR  EnableBusSupport=off
  S-Function1 : S-Function  FunctionName=sewer_asm1  Parameters=ASM1_SEWERINIT, ASM1_PARS, SPAR  EnableBusSupport=off
  S-Function2 : S-Function  FunctionName=sewer_asm1  Parameters=ASM1_SEWERINIT, ASM1_PARS, SPAR  EnableBusSupport=off
  Selector9 : Selector  InputPortWidth=22  IndexOptions=Index vector (dialog)  Indices=[1 2 3 4 5 6 7 8 9 10 11 12 13 14 15 16 17 18 19 20 21]  OutputSizes=1
  Out1 : Outport
  wires:
  S-Function/1 -> S-Function1/1
  S-Function1/1 -> S-Function2/1
  S-Function2/1 -> Selector9/1
  Mux1/1 -> S-Function/1
  Constant/1 -> Mux1/2
  In1/1 -> Mux1/1
  Selector9/1 -> Out1/1

== system ASM1_Influentmodel/ASM1/sewer/sewer4 ==
  In1 : Inport
  Constant : Constant
  Mux1 : Mux  Inputs=2
  S-Function : S-Function  FunctionName=sewer_asm1  Parameters=ASM1_SEWERINIT, ASM1_PARS, SPAR  EnableBusSupport=off
  S-Function1 : S-Function  FunctionName=sewer_asm1  Parameters=ASM1_SEWERINIT, ASM1_PARS, SPAR  EnableBusSupport=off
  S-Function2 : S-Function  FunctionName=sewer_asm1  Parameters=ASM1_SEWERINIT, ASM1_PARS, SPAR  EnableBusSupport=off
  Selector9 : Selector  InputPortWidth=22  IndexOptions=Index vector (dialog)  Indices=[1 2 3 4 5 6 7 8 9 10 11 12 13 14 15 16 17 18 19 20 21]  OutputSizes=1
  Out1 : Outport
  wires:
  S-Function/1 -> S-Function1/1
  S-Function1/1 -> S-Function2/1
  S-Function2/1 -> Selector9/1
  Mux1/1 -> S-Function/1
  Constant/1 -> Mux1/2
  In1/1 -> Mux1/1
  Selector9/1 -> Out1/1

== system ASM1_Influentmodel/ASM1/sewer/sewer5 ==
  In1 : Inport
  Constant : Constant
  Mux1 : Mux  Inputs=2
  S-Function : S-Function  FunctionName=sewer_asm1  Parameters=ASM1_SEWERINIT, ASM1_PARS, SPAR  EnableBusSupport=off
  S-Function1 : S-Function  FunctionName=sewer_asm1  Parameters=ASM1_SEWERINIT, ASM1_PARS, SPAR  EnableBusSupport=off
  S-Function2 : S-Function  FunctionName=sewer_asm1  Parameters=ASM1_SEWERINIT, ASM1_PARS, SPAR  EnableBusSupport=off
  Selector9 : Selector  InputPortWidth=22  IndexOptions=Index vector (dialog)  Indices=[1 2 3 4 5 6 7 8 9 10 11 12 13 14 15 16 17 18 19 20 21]  OutputSizes=1
  Out1 : Outport
  wires:
  S-Function/1 -> S-Function1/1
  S-Function1/1 -> S-Function2/1
  S-Function2/1 -> Selector9/1
  Mux1/1 -> S-Function/1
  Constant/1 -> Mux1/2
  In1/1 -> Mux1/1
  Selector9/1 -> Out1/1

== system ASM1_Influentmodel/ASM1/sewer/sewer6 ==
  In1 : Inport
  Constant : Constant
  Mux1 : Mux  Inputs=2
  S-Function : S-Function  FunctionName=sewer_asm1  Parameters=ASM1_SEWERINIT, ASM1_PARS, SPAR  EnableBusSupport=off
  S-Function1 : S-Function  FunctionName=sewer_asm1  Parameters=ASM1_SEWERINIT, ASM1_PARS, SPAR  EnableBusSupport=off
  S-Function2 : S-Function  FunctionName=sewer_asm1  Parameters=ASM1_SEWERINIT, ASM1_PARS, SPAR  EnableBusSupport=off
  Selector9 : Selector  InputPortWidth=22  IndexOptions=Index vector (dialog)  Indices=[1 2 3 4 5 6 7 8 9 10 11 12 13 14 15 16 17 18 19 20 21]  OutputSizes=1
  Out1 : Outport
  wires:
  S-Function/1 -> S-Function1/1
  S-Function1/1 -> S-Function2/1
  S-Function2/1 -> Selector9/1
  Mux1/1 -> S-Function/1
  Constant/1 -> Mux1/2
  In1/1 -> Mux1/1
  Selector9/1 -> Out1/1

== system ASM1_Influentmodel/ASM1/sewer/sewer7 ==
  In1 : Inport
  Constant : Constant
  Mux1 : Mux  Inputs=2
  S-Function : S-Function  FunctionName=sewer_asm1  Parameters=ASM1_SEWERINIT, ASM1_PARS, SPAR  EnableBusSupport=off
  S-Function1 : S-Function  FunctionName=sewer_asm1  Parameters=ASM1_SEWERINIT, ASM1_PARS, SPAR  EnableBusSupport=off
  S-Function2 : S-Function  FunctionName=sewer_asm1  Parameters=ASM1_SEWERINIT, ASM1_PARS, SPAR  EnableBusSupport=off
  Selector9 : Selector  InputPortWidth=22  IndexOptions=Index vector (dialog)  Indices=[1 2 3 4 5 6 7 8 9 10 11 12 13 14 15 16 17 18 19 20 21]  OutputSizes=1
  Out1 : Outport
  wires:
  S-Function/1 -> S-Function1/1
  S-Function1/1 -> S-Function2/1
  S-Function2/1 -> Selector9/1
  Mux1/1 -> S-Function/1
  Constant/1 -> Mux1/2
  In1/1 -> Mux1/1
  Selector9/1 -> Out1/1

== system ASM1_Influentmodel/ASM1/sewer/sewer8 ==
  In1 : Inport
  Constant : Constant
  Mux1 : Mux  Inputs=2
  S-Function : S-Function  FunctionName=sewer_asm1  Parameters=ASM1_SEWERINIT, ASM1_PARS, SPAR  EnableBusSupport=off
  S-Function1 : S-Function  FunctionName=sewer_asm1  Parameters=ASM1_SEWERINIT, ASM1_PARS, SPAR  EnableBusSupport=off
  S-Function2 : S-Function  FunctionName=sewer_asm1  Parameters=ASM1_SEWERINIT, ASM1_PARS, SPAR  EnableBusSupport=off
  Selector9 : Selector  InputPortWidth=22  IndexOptions=Index vector (dialog)  Indices=[1 2 3 4 5 6 7 8 9 10 11 12 13 14 15 16 17 18 19 20 21]  OutputSizes=1
  Out1 : Outport
  wires:
  S-Function/1 -> S-Function1/1
  S-Function1/1 -> S-Function2/1
  S-Function2/1 -> Selector9/1
  Mux1/1 -> S-Function/1
  Constant/1 -> Mux1/2
  In1/1 -> Mux1/1
  Selector9/1 -> Out1/1
